simulink model "ur_mex_demo"  (R2023b)
settings: Solver=FixedStepAuto  StartTime=0.0  StopTime=80  FixedStep=0.01  RelTol=1e-3
settings Model: Creator=Gavin  LastModifiedBy=Gavin

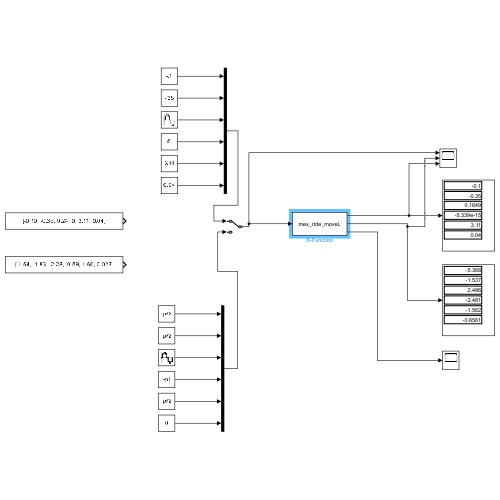
[thumbnail: Simulink's stored preview of the top-level diagram]
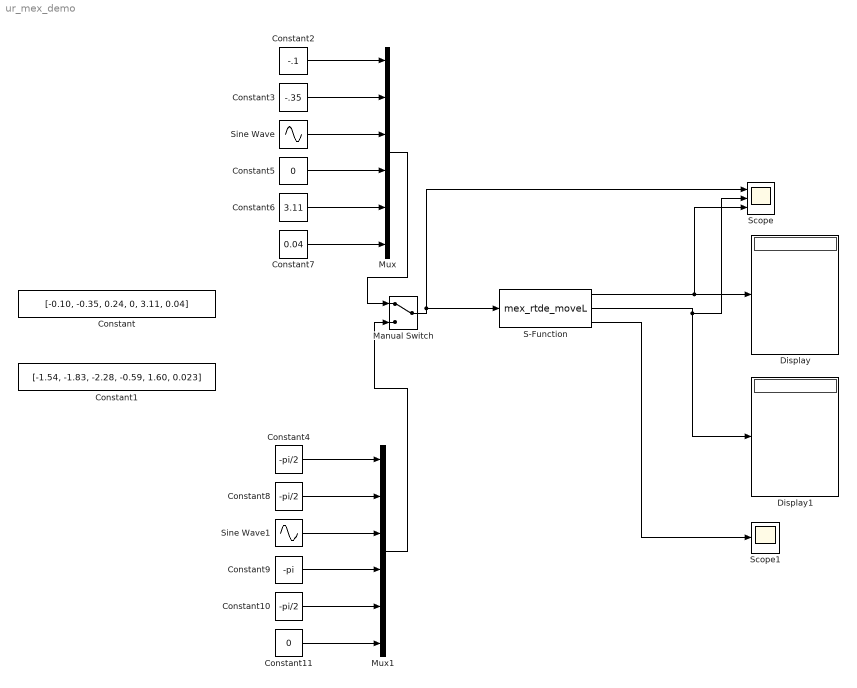
== system ur_mex_demo ==
  Constant : Constant  Value=[-0.10, -0.35, 0.24, 0, 3.11, 0.04]
  Constant1 : Constant  Value=[-1.54, -1.83, -2.28, -0.59, 1.60, 0.023]
  Constant10 : Constant  Value=-pi/2
  Constant11 : Constant  Value=0
  Constant2 : Constant  Value=-.1
  Constant3 : Constant  Value=-.35
  Constant4 : Constant  Value=-pi/2
  Constant5 : Constant  Value=0
  Constant6 : Constant  Value=3.11
  Constant7 : Constant  Value=0.04
  Constant8 : Constant  Value=-pi/2
  Constant9 : Constant  Value=-pi
  Display : Display
  Display1 : Display
  Manual Switch : ManualSwitch
  Mux : Mux  Inputs=6
  Mux1 : Mux  Inputs=6
  S-Function : S-Function  FunctionName=mex_rtde_moveL  Parameters=3 5 0.05 '192.168.255.128'  SFunctionDeploymentMode=off  EnableBusSupport=off
  Scope : Scope  NumInputPorts=3
  Scope1 : Scope
  Sine Wave : Sin  Amplitude=.1  Bias=.2  SampleTime=0.01
  Sine Wave1 : Sin  Amplitude=pi/4  Bias=pi/2  SampleTime=0.01
  wires:
  S-Function/1 -> Display/1, Scope/3
  Manual Switch/1 -> Scope/1, S-Function/1
  Constant7/1 -> Mux/6
  Constant6/1 -> Mux/5
  Constant5/1 -> Mux/4
  Constant3/1 -> Mux/2
  Constant2/1 -> Mux/1
  Sine Wave/1 -> Mux/3
  Sine Wave1/1 -> Mux1/3
  Constant4/1 -> Mux1/1
  Constant8/1 -> Mux1/2
  Constant9/1 -> Mux1/4
  Constant10/1 -> Mux1/5
  Constant11/1 -> Mux1/6
  Mux/1 -> Manual Switch/1
  Mux1/1 -> Manual Switch/2
  S-Function/2 -> Display1/1, Scope/2
  S-Function/3 -> Scope1/1
